simulink model "QuarterCarPowerGen"  (R2020a)
settings: Solver=VariableStepAuto  StartTime=0.0  StopTime=10.0  RelTol=1e-3
settings Model: Creator=Aditya Sharma  LastModifiedBy=Aditya Sharma

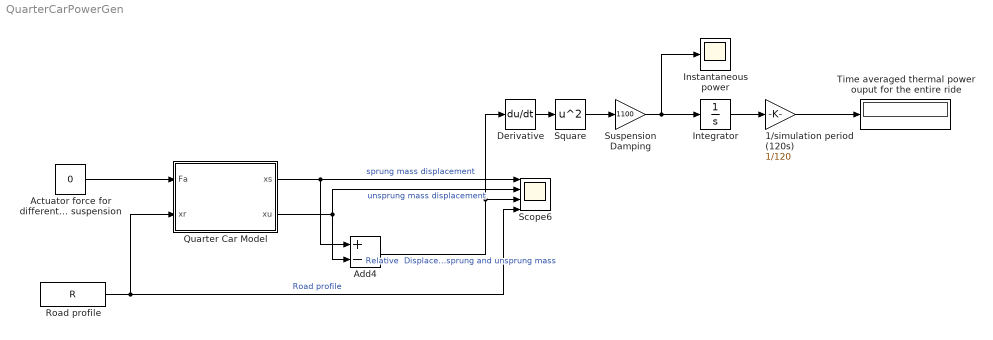
== system QuarterCarPowerGen ==
  1/simulation period (120s) : Gain  Gain=1/120
  "Actuator force for different types of suspension " : Constant  Value=0
  Add4 : Sum  Inputs=+-
  Derivative : Derivative
  "Instantaneous power " : Scope
  Integrator : Integrator
  Quarter Car Model : Subsystem
  "Road profile " : FromWorkspace  VariableName=R
  Scope6 : Scope  NumInputPorts=4
  Square : Math  Operator=square  SaturateOnIntegerOverflow=on
  Suspension Damping : Gain  Gain=1100
  "Time averaged thermal power ouput for the entire ride " : Display
  wires:
  1/simulation period (120s)/1 -> "Time averaged thermal power ouput for the entire ride "/1
  Add4/1 -> Derivative/1, Scope6/3  "Relative  Displacement b/w sprung and unsprung mass"
  Suspension Damping/1 -> "Instantaneous power "/1, Integrator/1
  "Actuator force for different types of suspension "/1 -> Quarter Car Model/1(Fa)
  Square/1 -> Suspension Damping/1
  Integrator/1 -> 1/simulation period (120s)/1
  "Road profile "/1 -> Quarter Car Model/2(xr), Scope6/4  "Road profile"
  Quarter Car Model/1(xs) -> Add4/1, Scope6/1  "sprung mass displacement"
  Derivative/1 -> Square/1
  Quarter Car Model/2(xu) -> Scope6/2, Add4/2  "unsprung mass displacement"

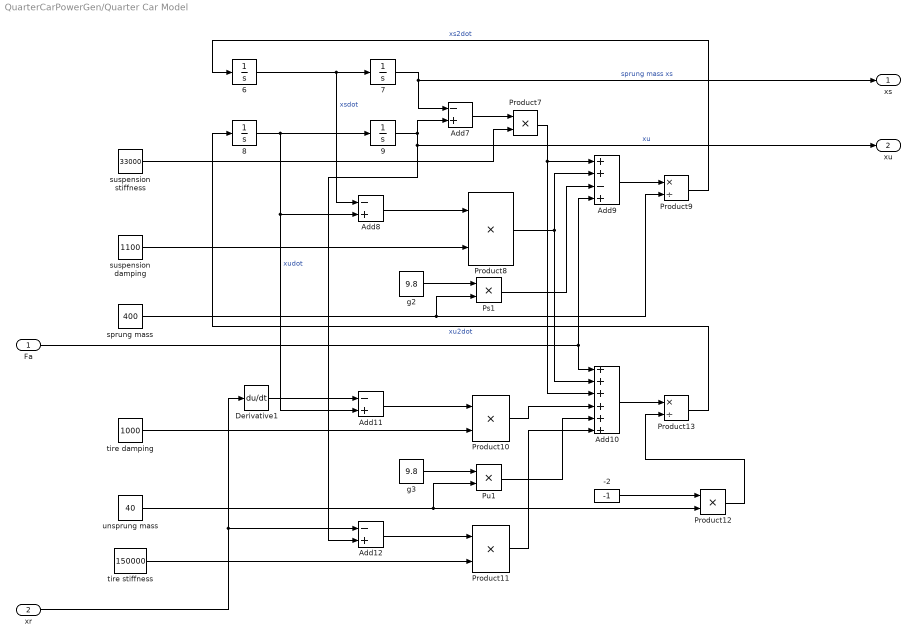
== system QuarterCarPowerGen/Quarter Car Model ==
  Fa : Inport
  xr : Inport  Port=2
  -2 : Constant  Value=-1
  {6..9} (4 alike) : Integrator
  Add10 : Sum  Inputs=++++++
  Add{7..8,11..12} (4 alike) : Sum  Inputs=-+
  Add9 : Sum  Inputs=++-+
  Derivative1 : Derivative
  Product{7..8,10..12} (5 alike) : Product
  Product13 : Product  Inputs=*/
  Product9 : Product  Inputs=*/
  Ps1 : Product
  Pu1 : Product
  g2 : Constant  Value=9.8
  g3 : Constant  Value=9.8
  sprung mass : Constant  Value=400
  suspension damping : Constant  Value=1100
  suspension stiffness : Constant  Value=33000
  "tire damping " : Constant  Value=1000
  tire stiffness : Constant  Value=150000
  unsprung mass : Constant  Value=40
  xs : Outport
  xu : Outport  Port=2
  wires:
  g2/1 -> Ps1/1
  Product12/1 -> Product13/2
  g3/1 -> Pu1/1
  Ps1/1 -> Add9/3
  Add10/1 -> Product13/1
  -2/1 -> Product12/1
  unsprung mass/1 -> Pu1/2, Product12/2
  Product11/1 -> Add10/6
  Add12/1 -> Product11/1
  tire stiffness/1 -> Product11/2
  xr/1 -> Add12/1, Derivative1/1
  Pu1/1 -> Add10/5
  Product10/1 -> Add10/4
  Add11/1 -> Product10/1
  "tire damping "/1 -> Product10/2
  Derivative1/1 -> Add11/1
  sprung mass/1 -> Product9/2, Ps1/2
  Add9/1 -> Product9/1
  Fa/1 -> Add10/1, Add9/4
  Product8/1 -> Add10/2, Add9/2
  Product7/1 -> Add10/3, Add9/1
  suspension damping/1 -> Product8/2
  Add8/1 -> Product8/1
  suspension stiffness/1 -> Product7/2
  Add7/1 -> Product7/1
  9/1 -> Add12/2, xu/1, Add7/2  "xu"
  Product13/1 -> 8/1  "xu2dot"
  8/1 -> 9/1, Add8/2, Add11/2  "xudot"
  7/1 -> Add7/1, xs/1  "sprung mass xs"
  Product9/1 -> 6/1  "xs2dot"
  6/1 -> 7/1, Add8/1  "xsdot"
